simulink model "Taijia_Model"  (R2014b)
settings: Solver=ode45  StartTime=0.0  StopTime=5  RelTol=1e-3
values from neighbouring files (symbols this model uses):
  m2 = input(1,1)    [AdaptFunc.m]
  P0 = input(1,2)    [AdaptFunc.m]
undefined symbols (not defined in the file or in its folder): zhifanliju, zhongliju
settings Model: Creator=Administrator  LastModifiedBy=wuqiankang
settings DebuggingCC: SolverPrmCheckMsg=none

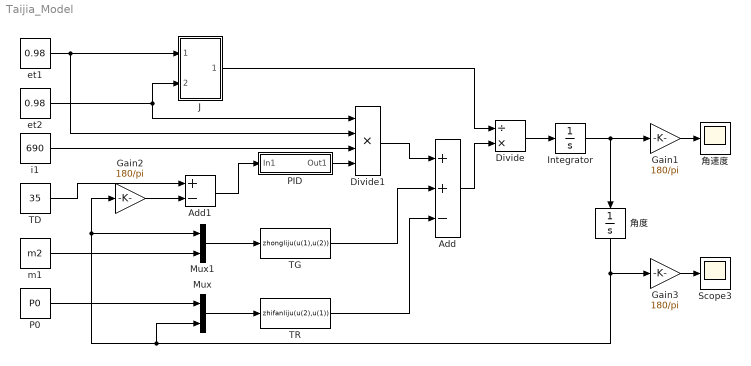
== system Taijia_Model ==
  Add : Sum  Inputs=++-
  Add1 : Sum  Inputs=+-
  Divide : Product  Inputs=/*
  Divide1 : Product  Inputs=****
  Gain1 : Gain  Gain=180/pi
  Gain2 : Gain  Gain=180/pi
  Gain3 : Gain  Gain=180/pi
  Integrator : Integrator
  J : Subsystem
  Mux : Mux  Inputs=2
  Mux1 : Mux  Inputs=2
  "P0 " : Constant  Value=P0
  PID : Subsystem
  Scope3 : Scope
      settings: TimeRange=1.5  YMin=0  YMax=40  SaveName=jiaodu
  TD : Constant  Value=35
  TG : MATLABFcn  MATLABFcn=zhongliju(u(1),u(2))
  "TR " : MATLABFcn  MATLABFcn=zhifanliju(u(2),u(1))  Output1D=off
  et1 : Constant  Value=0.98
  et2 : Constant  Value=0.98
  i1 : Constant  Value=690
  "m1 " : Constant  Value=m2
  角度 : Integrator
  角速度 : Scope
      settings: SaveName=jiaosudu  DataFormat=Structure
  wires:
  TG/1 -> Add/2
  "TR "/1 -> Add/3
  Divide/1 -> Integrator/1
  角度/1 -> Gain3/1, Mux/2, Gain2/1, Mux1/1
  et1/1 -> Divide1/2, J/1(In1)
  et2/1 -> J/2(In2), Divide1/1
  J/1(Out1) -> Divide/1
  TD/1 -> Add1/1
  Add1/1 -> PID/1(In1)
  Gain1/1 -> 角速度/1
  Integrator/1 -> Gain1/1, 角度/1
  Gain2/1 -> Add1/2
  Add/1 -> Divide/2
  Gain3/1 -> Scope3/1
  i1/1 -> Divide1/3
  Divide1/1 -> Add/1
  PID/1(Out1) -> Divide1/4
  Mux/1 -> "TR "/1
  "P0 "/1 -> Mux/1
  Mux1/1 -> TG/1
  "m1 "/1 -> Mux1/2

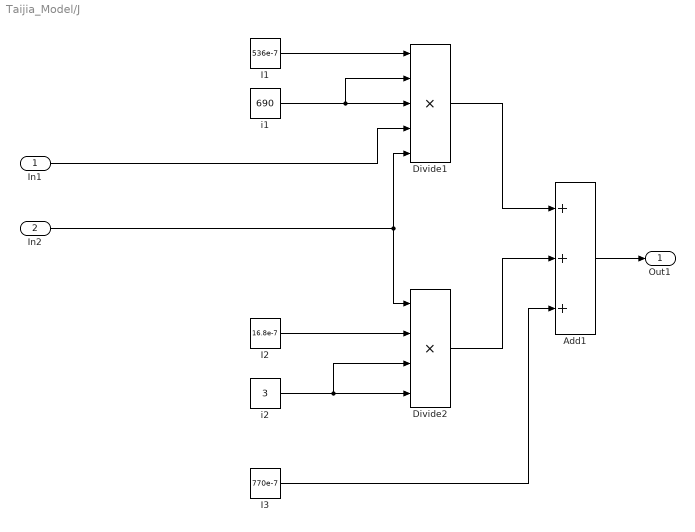
== system Taijia_Model/J ==
  In1 : Inport
  In2 : Inport  Port=2
  Add1 : Sum  Inputs=+++
  Divide1 : Product  Inputs=*****
  Divide2 : Product  Inputs=****
  I1 : Constant  Value=536e-7
  I2 : Constant  Value=16.8e-7
  I3 : Constant  Value=770e-7
  i1 : Constant  Value=690
  i2 : Constant  Value=3
  Out1 : Outport
  wires:
  Divide2/1 -> Add1/2
  Divide1/1 -> Add1/1
  I3/1 -> Add1/3
  I2/1 -> Divide2/2
  Add1/1 -> Out1/1
  In2/1 -> Divide2/1, Divide1/5
  I1/1 -> Divide1/1
  i2/1 -> Divide2/3, Divide2/4
  In1/1 -> Divide1/4
  i1/1 -> Divide1/3, Divide1/2

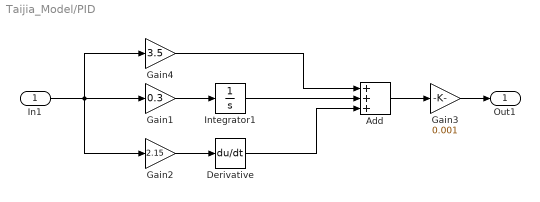
== system Taijia_Model/PID ==
  In1 : Inport
  Add : Sum  Inputs=+++
  Derivative : Derivative
  Gain1 : Gain  Gain=0.3
  Gain2 : Gain  Gain=2.15
  Gain3 : Gain  Gain=0.001
  Gain4 : Gain  Gain=3.5
  Integrator1 : Integrator
  Out1 : Outport
  wires:
  Gain4/1 -> Add/1
  Derivative/1 -> Add/3
  In1/1 -> Gain4/1, Gain2/1, Gain1/1
  Integrator1/1 -> Add/2
  Add/1 -> Gain3/1
  Gain2/1 -> Derivative/1
  Gain1/1 -> Integrator1/1
  Gain3/1 -> Out1/1
